simulink model "MotorUNDReifenV2"  (R2024a)
settings: Solver=VariableStepAuto  StartTime=0.0  StopTime=10.0  RelTol=1e-3
values from neighbouring files (symbols this model uses):
  A_neu = [0 1 0; 0 A22 A23; 0 A32 A33]    [Parameter.m]
  B_neu = [0; 0; 1/motorinductivity]    [Parameter.m]
  CT_i = [0 0 1]    [Parameter.m]
  CT_omega = [0 1 0]    [Parameter.m]
  E_neu = [0; -((m_last/2 + m_Reifen) / (motorinertia + (m_Reifen *Reifen_Radius^2)/50) * g * mue * Reifen_Radius); 0 ]    [Parameter.m]
  Motoruebersetzung = 100    [Model1Sensibilities.m]    (also in Model1numericalPSA.m; Model2Sensibilities.m; Modellvalidierung.m; MotorSens2.m)
  x0_neu = [0; 0.01; 0]    [Parameter.m]
settings Model: Creator=jakob  LastModifiedBy=jakob

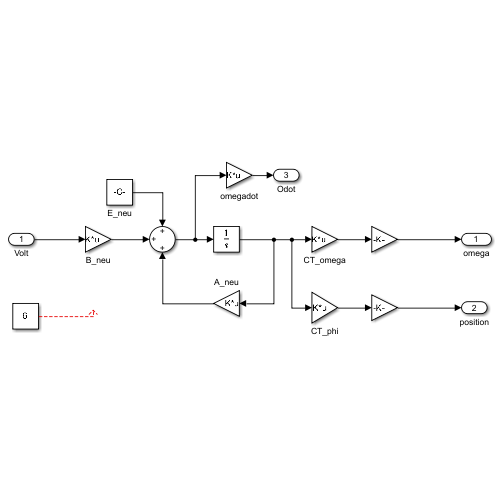
[thumbnail: Simulink's stored preview of the top-level diagram]
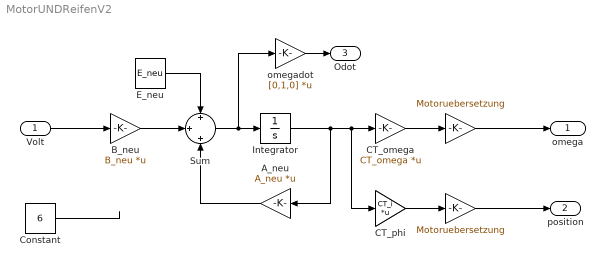
== system MotorUNDReifenV2 ==
  Volt : Inport
  " " : Gain  Gain=Motoruebersetzung
  "  " : Gain  Gain=Motoruebersetzung
  A_neu : Gain  Gain=A_neu  Multiplication=Matrix(K*u)
  B_neu : Gain  Gain=B_neu  Multiplication=Matrix(K*u)
  CT_omega : Gain  Gain=CT_omega  Multiplication=Matrix(K*u)
  CT_phi : Gain  Gain=CT_i  Multiplication=Matrix(K*u)
  Constant : Constant  Value=6
  E_neu : Constant  Value=E_neu
  Integrator : Integrator  InitialCondition=x0_neu
  Sum : Sum  Inputs=+|+|+
  omegadot : Gain  Gain=[0,1,0]  Multiplication=Matrix(K*u)
  omega : Outport
  position : Outport  Port=2
  Odot : Outport  Port=3
  wires:
  Constant/1 -> ?
  " "/1 -> position/1
  "  "/1 -> omega/1
  CT_omega/1 -> "  "/1
  Volt/1 -> B_neu/1
  Integrator/1 -> CT_phi/1, CT_omega/1, A_neu/1
  Sum/1 -> omegadot/1, Integrator/1
  CT_phi/1 -> " "/1
  E_neu/1 -> Sum/1
  B_neu/1 -> Sum/2
  A_neu/1 -> Sum/3
  omegadot/1 -> Odot/1
